simulink model "tvc_ppj"  (R2025a)
settings: Solver=VariableStepAuto  StartTime=0.0  StopTime=10.0  RelTol=1e-3
libraries: simulink_extras x2, slpidlib x1
settings Model: Creator=pjpra  LastModifiedBy=pjpra

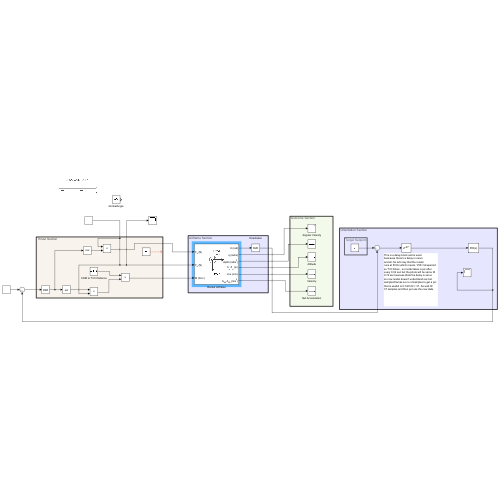
[thumbnail: Simulink's stored preview of the top-level diagram]
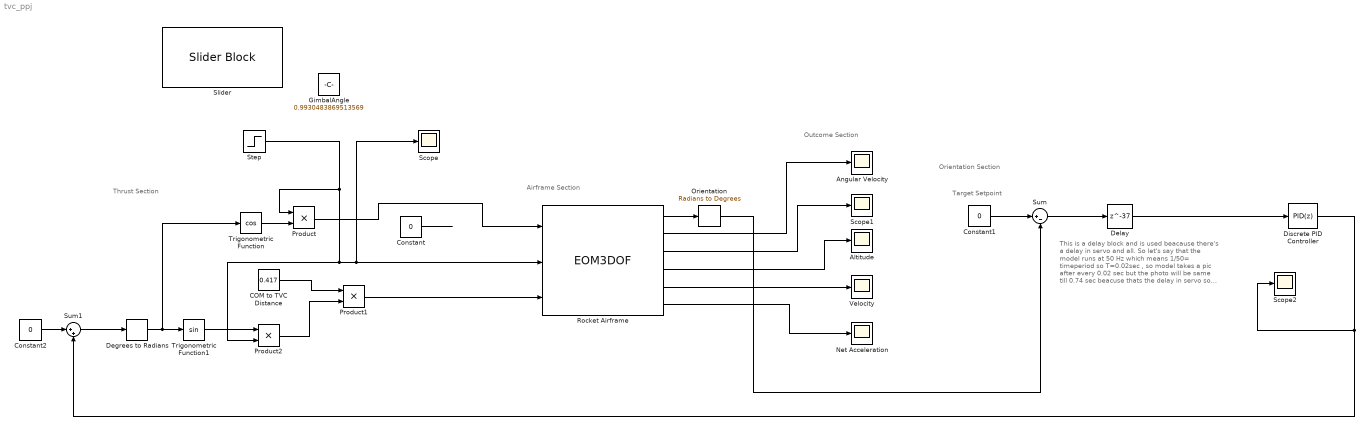
== system tvc_ppj ==
  note: Orientation Section
  note: Thrust Section
  note: This is a delay block and is used
      | beacause there's a delay in servo
      | and all. So let's say that the model
      | runs at 50 Hz which means 1/50= timeperiod
      | so T=0.02sec , so model takes a pic after
      | every 0.02 sec but the photo will be same till
      | 0.74 sec beacuse thats the delay in servo
      | so now model doesn't understand sec but
      | samples/frames so no of samples to get a pic
      | that is usefull is 0.74/0.02 = 37. So wait till
      | 37 samples and then put use the new data.
  note: Target Setpoint
  note: Outcome Section
  note: Airframe Section
  Altitude : Scope
      settings: ActiveDisplayYMinimum=-721.743314014895  ActiveDisplayYMaximum=1205.5291641351232  DataLoggingVariableName=ScopeData3
  Angular Velocity : Scope
      settings: ActiveDisplayYMinimum=-0.11876162628360287  ActiveDisplayYMaximum=0.0030873397763223898
  COM to TVC Distance : Constant  Value=0.417
  Constant : Constant  Value=0
  Constant1 : Constant  Value=0
  Constant2 : Constant  Value=0
  Degrees to Radians : simulink_extras/Transformations/Degrees to Radians
  Delay : Delay  DelayLength=37
  Discrete PID Controller : slpidlib/PID Controller  Controller=PID  Form=Parallel  TimeDomain=Discrete-time  UseExternalTs=off  SampleTime=0.02  IntegratorMethod=Forward Euler  FilterMethod=Forward Euler  ControllerParametersSource=internal  P=0.7  I=0.17  UseKiTs=off  D=0.15  UseExternalDerivativeSource=off  N=100  UseFilter=on  TunerSelectOption=Transfer Function Based (PID Tuner App)  InitialConditionSource=internal  InitialConditionForIntegrator=0  InitialConditionForFilter=0  DifferentiatorICPrevScaledInput=0  ExternalReset=none  TrackingMode=off  Kt=1  LimitOutput=off  SatLimitsSource=internal  UpperSaturationLimit=inf  LowerSaturationLimit=-inf  LinearizeAsGain=off  AntiWindupMode=none  Kb=1  LimitIntegrator=off  UpperIntegratorSaturationLimit=inf  LowerIntegratorSaturationLimit=-inf  POutMin=[]  POutMax=[]  IOutMin=[]  IOutMax=[]  DOutMin=[]  DOutMax=[]  NOutMin=[]  NOutMax=[]  SumOutMin=[]  SumOutMax=[]  SaturationOutMin=[]  SaturationOutMax=[]  PParamMin=[]  PParamMax=[]  IParamMin=[]  IParamMax=[]  DParamMin=[]  DParamMax=[]  NParamMin=[]  NParamMax=[]  KbParamMin=[]  KbParamMax=[]  KtParamMin=[]  KtParamMax=[]  KbOutMin=[]  KbOutMax=[]  KtOutMin=[]  KtOutMax=[]  IntegratorOutMin=[]  IntegratorOutMax=[]  FilterOutMin=[]  FilterOutMax=[]  SumI1OutMin=[]  SumI1OutMax=[]  SumI2OutMin=[]  SumI2OutMax=[]  SumI3OutMin=[]  SumI3OutMax=[]  SumI4OutMin=[]  SumI4OutMax=[]  SumDOutMin=[]  SumDOutMax=[]  DifferentiatorOutMin=[]  DifferentiatorOutMax=[]  FilterDiffOutCoefMin=[]  FilterDiffOutCoefMax=[]  ReciprocalOutMin=[]  ReciprocalOutMax=[]  SumDenOutMin=[]  SumDenOutMax=[]  SumNumOutMin=[]  SumNumOutMax=[]  DivideOutMin=[]  DivideOutMax=[]  UdiffTsProdOutMin=[]  UdiffTsProdOutMax=[]  NTsProdOutMin=[]  NTsProdOutMax=[]  UintegralTsProdOutMin=[]  UintegralTsProdOutMax=[]  UngainTsProdOutMin=[]  UngainTsProdOutMax=[]  ClampingZeroOutDataTypeStr=Inherit: Inherit via back propagation  ClampingZeroOutMin=[]  ClampingZeroOutMax=[]  FilterDenConstantOutDataTypeStr=Inherit: Inherit via back propagation  FilterDenConstantOutMin=[]  FilterDenConstantOutMax=[]  PCopyOutDataTypeStr=Inherit: Inherit via back propagation  PCopyOutMin=[]  PCopyOutMax=[]  NCopyOutDataTypeStr=Inherit: Inherit via back propagation  NCopyOutMin=[]  NCopyOutMax=[]  IntegratorContinuousStateAttributes=''  IntegratorStateMustResolveToSignalObject=off  IntegratorRTWStateStorageClass=Auto  FilterContinuousStateAttributes=''  FilterStateMustResolveToSignalObject=off  FilterRTWStateStorageClass=Auto  ParallelPVariant=InternalParameters  IdealPVariant=Disabled  IVariant=InternalParameters  DVariant=InternalParameters  IntegratorVariant=Discrete  SatVariant=Disabled  AWVariant=Passthrough  PCopyVariant=Disabled  TRVariant=Disabled  FdbkBlocksVariant=Forward  IdealPFdbkVariant=Disabled  SatFdbkVariant=Disabled  DerivativeFilterVariant=ForwardEulerFilter  NVariant=InternalParameters  NCopyVariant=Disabled  FilterICVariant=InternalICsFilter  IntegratorICVariant=InternalICs  ExternalResetVariant=Disabled  TRSumVariant=Passthrough  SumFdbkVariant=Disabled  SumVariant=Sum_PID  TsampFilterVariant=InternalTs  TsampNgainVariant=Passthrough  TsampIntegralVariant=Disabled_SignalSpec  ExternalSaturationOutDataTypeStr=Inherit: Same as second input  DerivativeSourceVariant=ErrorSignal  PreIntVariant=InternalPreInt
      settings: LibrarySourceBlock=simulink/Discrete/Discrete PID Controller
  GimbalAngle : Constant  Value=0.9930483869513569
  Net Acceleration : Scope
      settings: DataLoggingVariableName=ScopeData5
  "Orientation " : simulink_extras/Transformations/Radians to Degrees
  Product : Product
  Product1 : Product
  Product2 : Product
  Rocket Airframe : EOM3DOF  theta_ini=0.0174533*3  mass=0.654  Iyy=0.07651  g=-9.81
  Scope : Scope
  Scope1 : Scope
      settings: DataLoggingVariableName=ScopeData2
  Scope2 : Scope
      settings: ActiveDisplayYMinimum=-487.00009113944532  ActiveDisplayYMaximum=410.01516266039914  DataLoggingVariableName=ScopeData6
  Slider : SliderBlock  ScaleMin=-1  ScaleMax=1  TickInterval=1
  Step : Step  Before=1  After=0  SampleTime=0
  Sum : Sum  Inputs=|+-
  Sum1 : Sum  Inputs=|++
  Trigonometric Function : Trigonometry  Operator=cos
  Trigonometric Function1 : Trigonometry
  Velocity : Scope
      settings: DataLoggingVariableName=ScopeData4
  wires:
  Constant/1 -> ?
  Trigonometric Function/1 -> Product/2
  COM to TVC Distance/1 -> Product1/1
  Product2/1 -> Product1/2
  Rocket Airframe/1 -> "Orientation "/1
  Step/1 -> Product/1, Product2/2, Scope/1, Rocket Airframe/2
  Trigonometric Function1/1 -> Product2/1
  Degrees to Radians/1 -> Trigonometric Function1/1, Trigonometric Function/1
  Rocket Airframe/2 -> Angular Velocity/1
  Rocket Airframe/3 -> Scope1/1
  Rocket Airframe/4 -> Altitude/1
  Rocket Airframe/5 -> Velocity/1
  Rocket Airframe/6 -> Net Acceleration/1
  "Orientation "/1 -> Sum/2
  Constant1/1 -> Sum/1
  Sum/1 -> Delay/1
  Delay/1 -> Discrete PID Controller/1
  Discrete PID Controller/1 -> Scope2/1, Sum1/2
  Constant2/1 -> Sum1/1
  Sum1/1 -> Degrees to Radians/1
  Product1/1 -> Rocket Airframe/3
  Product/1 -> Rocket Airframe/1
